simulink model "kwta2_block"  (R2024b)
settings: Solver=VariableStepAuto  StartTime=0.0  StopTime=2e-5  RelTol=1e-3
libraries: fl_lib x104, ee_lib x58, nesl_utility x13
(part 1 of 2)
settings Model: Creator=xyl  LastModifiedBy=James
settings SolverCC: AlgebraicLoopSolver=TrustRegion
settings DataIOCC: ReturnWorkspaceOutputs=off
settings DebuggingCC: UnconnectedInputMsg=warning  UnconnectedOutputMsg=warning  UnconnectedLineMsg=warning  ArithmeticOperatorsInVariantConditions=warning
settings ModelReferenceCC: EnableRefExpFcnMdlSchedulingChecks=on
settings SFSimCC: CustomCodeUndefinedFunction=UseInterfaceOnly
settings RTWCC: GPUComputeCapability=3.5

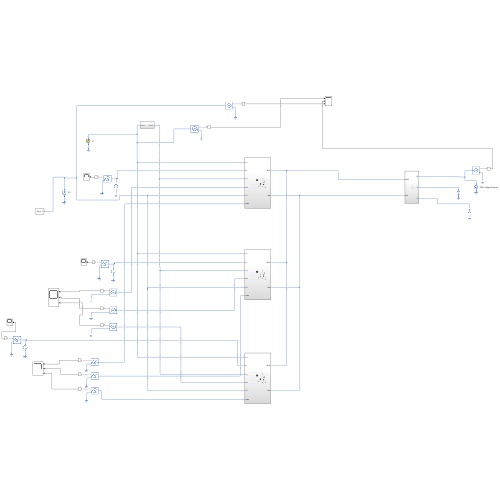
[thumbnail: Simulink's stored preview of the top-level diagram]
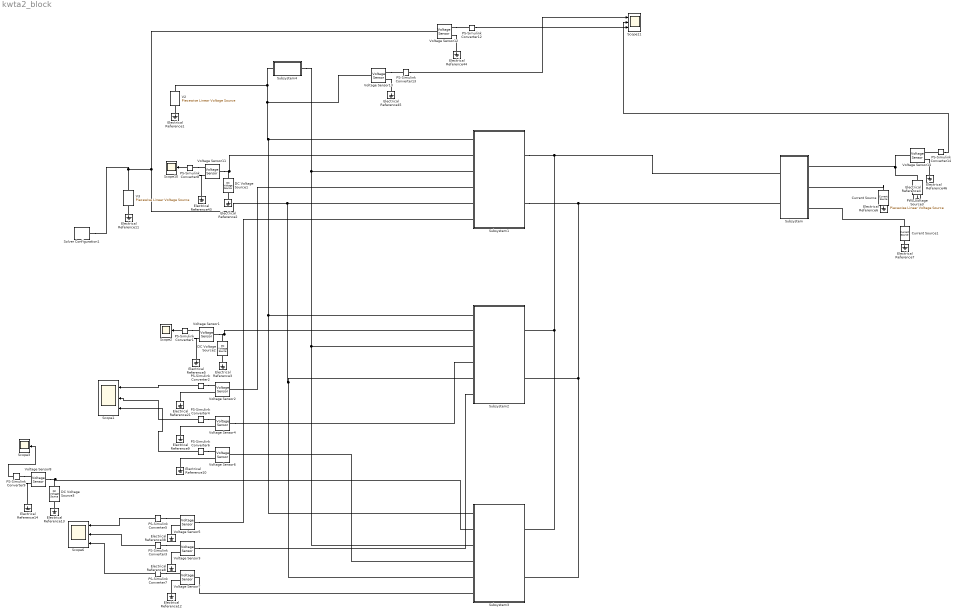
== system kwta2_block ==
  Current Source : ee_lib/Sources/Current Source  dc_current=40 uA  ac_current=0 A  ac_shift=0 rad  ac_frequency=60 Hz  noise_mode=0  PSD=0 A^2/Hz  sample_time=1e-3 s  repeatability=1  user_seed=0  auto_seed=3686359230  i_specify=off  i_priority=None  i=0 A  i_nominal_specify=off  i_nominal_value=1  i_nominal_unit=A  v_specify=off  v_priority=None  v=0 V  v_nominal_specify=off  v_nominal_value=1  v_nominal_unit=V
  Current Source1 : ee_lib/Sources/Current Source  dc_current=20 uA  ac_current=0 A  ac_shift=0 rad  ac_frequency=60 Hz  noise_mode=0  PSD=0 A^2/Hz  sample_time=1e-3 s  repeatability=1  user_seed=0  auto_seed=98181336  i_specify=off  i_priority=None  i=0 A  i_nominal_specify=off  i_nominal_value=1  i_nominal_unit=A  v_specify=off  v_priority=None  v=0 V  v_nominal_specify=off  v_nominal_value=1  v_nominal_unit=V
  DC Voltage Source1 : fl_lib/Electrical/Electrical Sources/DC Voltage Source  v0=0.1 V
  DC Voltage Source2 : fl_lib/Electrical/Electrical Sources/DC Voltage Source  v0=0.2 V
  DC Voltage Source3 : fl_lib/Electrical/Electrical Sources/DC Voltage Source  v0=0.3 V
  Electrical Reference{1..14,21,38,43..46} (20 alike) : fl_lib/Electrical/Electrical Elements/Electrical Reference
  PS-Simulink Converter{1..9,12..14} (12 alike) : nesl_utility/PS-Simulink Converter  PhysicalDomain=network_engine_domain  SubClassName=ps_output  LeftPortType=input  RightPortType=output  PseudoPeriodic=off  Frequencies=[]  VectorFormat=1-D array  Unit=1  AffineConversion=off
  PWL Voltage Source3 : ee_lib/Additional Components/SPICE Sources/Piecewise Linear Voltage Source  TIMElist=[0, 4, 4.01, 10, 10.01] us  VOLTlist=[0, 0, 5, 5, 5] V  INTERP=1  EXTRAP=2
      settings: InternalSimscapePortConfiguration="{\"Bottom\":[],\"Left\":[{\"id\":\"p\",\"label\":\"+\",\"type\":\"foundation.electrical.electrical\"}],\"Right\":[{\"id\":\"n\",\"label\":\"-\",\"type\":\"foundation.electrical.electrical\"}],\"Top\":[]}"
  Scope1 : Scope  NumInputPorts=3
  Scope10 : Scope
  Scope11 : Scope  NumInputPorts=3
  Scope2 : Scope
  Scope3 : Scope
  Scope6 : Scope  NumInputPorts=3
  Solver Configuration1 : nesl_utility/Solver Configuration  PhysicalDomain=network_engine_domain  SubClassName=solver  LeftPortType=input  RightPortType=generic  Tones=[]  Harmonics=[]  SimulateNoise=off  Profile=off  UseLocalSampling=off  EnableSwitchedLinearOptims=on  FrequencyDomain=off  UseCCode=off  RelTol=0.001  AbsTol=1e-06  MinStep=1e-09  ToWorkspace=off  RevertToSquareIcSolve=off  NumHomotopyIterations=100  PhasorMode=off  PhasorModeNumHarmonics=1  ConsistencySolver=NEWTON_FTOL  IndexReductionMethod=DerivativeReplacement  DoDC=on  ResidualTolerance=1e-09  ConsistencyTolSource=GLOBAL  ConsistencyAbsTol=0.001  ConsistencyRelTol=0.001  ConsistencyTolFactor=0.001  UseLocalSolver=on  LocalSolverChoice=NE_BACKWARD_EULER_ADVANCER  ResolveIndetEquations=on  FunctionEvalNumThread=1  LocalSolverSampleTime=1e-9  DoFixedCost=off  MaxNonlinIter=3  MaxModeIter=2  ComputeImpulses=off  ImpulseIterations=2  LinearAlgebra=Sparse  LinearAlgebraNumThread=0  EquationFormulation=NE_TIME_EF  DelaysMemoryBudget=1024  AutomaticFiltering=on  FilteringTimeConstant=0.01  PartitionStorageMethod=AS_NEEDED  PartitionMemoryBudget=1024  PartitionMethod=FAST  MultibodyUseLocalSolver=off  MultibodyLocalSolverChoice=ODE1  MultibodyLocalSolverSampleTime=0.001
  Subsystem : Subsystem
  Subsystem1 : Subsystem
  Subsystem2 : Subsystem
  Subsystem3 : Subsystem
  Subsystem4 : Subsystem
  V2 : ee_lib/Additional Components/SPICE Sources/Piecewise Linear Voltage Source  TIMElist=[0, 2, 2.01, 4, 4.1] us  VOLTlist=[0, 0, 5, 5, 5] V  INTERP=1  EXTRAP=2
      settings: InternalSimscapePortConfiguration="{\"Bottom\":[],\"Left\":[{\"id\":\"p\",\"label\":\"+\",\"type\":\"foundation.electrical.electrical\"}],\"Right\":[{\"id\":\"n\",\"label\":\"-\",\"type\":\"foundation.electrical.electrical\"}],\"Top\":[]}"
  V3 : ee_lib/Additional Components/SPICE Sources/Piecewise Linear Voltage Source  TIMElist=[0, 2, 14, 14.01, 16] us  VOLTlist=[0, 0, 0, 5, 5] V  INTERP=1  EXTRAP=2
      settings: InternalSimscapePortConfiguration="{\"Bottom\":[],\"Left\":[{\"id\":\"p\",\"label\":\"+\",\"type\":\"foundation.electrical.electrical\"}],\"Right\":[{\"id\":\"n\",\"label\":\"-\",\"type\":\"foundation.electrical.electrical\"}],\"Top\":[]}"
  Voltage Sensor{1..8,11..14} (12 alike) : fl_lib/Electrical/Electrical Sensors/Voltage Sensor
  wires:
  PS-Simulink Converter2/1 -> Scope1/1
  PS-Simulink Converter5/1 -> Scope6/1
  PS-Simulink Converter8/1 -> Scope10/1
  PS-Simulink Converter13/1 -> Scope11/1
  PS-Simulink Converter12/1 -> Scope11/3
  PS-Simulink Converter14/1 -> Scope11/2
  PS-Simulink Converter1/1 -> Scope2/1
  PS-Simulink Converter3/1 -> Scope6/2
  PS-Simulink Converter4/1 -> Scope1/2
  PS-Simulink Converter6/1 -> Scope1/3
  PS-Simulink Converter7/1 -> Scope6/3
  PS-Simulink Converter9/1 -> Scope3/1
  connections:
  Voltage Sensor11/LConn1 -- DC Voltage Source1/LConn1 -- Subsystem1/LConn2
  Electrical Reference1/LConn1 -- V2/RConn1
  Electrical Reference2/LConn1 -- DC Voltage Source1/RConn1
  Subsystem1/RConn1 -- Subsystem3/RConn1 -- Subsystem2/RConn1 -- Subsystem/LConn1
  Electrical Reference4/LConn1 -- PWL Voltage Source3/RConn1
  Electrical Reference6/LConn1 -- Current Source/RConn1
  Electrical Reference7/LConn1 -- Current Source1/RConn1
  Electrical Reference11/LConn1 -- V3/RConn1
  V3/LConn1 -- Solver Configuration1/RConn1 -- Voltage Sensor12/LConn1 -- Subsystem3/LConn5 -- Subsystem2/LConn5 -- Subsystem1/LConn5
  Voltage Sensor2/RConn2 -- Electrical Reference21/LConn1
  PS-Simulink Converter2/LConn1 -- Voltage Sensor2/RConn1
  Subsystem1/RConn2 -- Subsystem3/RConn2 -- Subsystem2/RConn2 -- Subsystem/LConn2
  Electrical Reference38/LConn1 -- Voltage Sensor5/RConn2
  PS-Simulink Converter5/LConn1 -- Voltage Sensor5/RConn1
  PS-Simulink Converter8/LConn1 -- Voltage Sensor11/RConn1
  Voltage Sensor11/RConn2 -- Electrical Reference43/LConn1
  Voltage Sensor12/RConn2 -- Electrical Reference44/LConn1
  Voltage Sensor12/RConn1 -- PS-Simulink Converter12/LConn1
  Voltage Sensor13/RConn2 -- Electrical Reference45/LConn1
  Voltage Sensor13/RConn1 -- PS-Simulink Converter13/LConn1
  Voltage Sensor14/RConn2 -- Electrical Reference46/LConn1
  PS-Simulink Converter14/LConn1 -- Voltage Sensor14/RConn1
  V2/LConn1 -- Subsystem4/RConn1 -- Subsystem3/LConn1 -- Subsystem2/LConn1 -- Subsystem1/LConn1 -- Voltage Sensor13/LConn1
  PWL Voltage Source3/LConn1 -- Voltage Sensor14/LConn1 -- Subsystem/RConn1
  Current Source/LConn1 -- Subsystem/RConn2
  Current Source1/LConn1 -- Subsystem/RConn3
  Subsystem4/LConn1 -- Subsystem3/LConn3 -- Subsystem2/LConn3 -- Subsystem1/LConn3
  Voltage Sensor5/LConn1 -- Subsystem1/LConn6
  Subsystem1/LConn4 -- Voltage Sensor2/LConn1
  Voltage Sensor1/LConn1 -- DC Voltage Source2/LConn1 -- Subsystem2/LConn2
  Voltage Sensor1/RConn2 -- Electrical Reference5/LConn1
  Electrical Reference3/LConn1 -- DC Voltage Source2/RConn1
  PS-Simulink Converter1/LConn1 -- Voltage Sensor1/RConn1
  PS-Simulink Converter3/LConn1 -- Voltage Sensor3/RConn1
  Electrical Reference8/LConn1 -- Voltage Sensor3/RConn2
  Voltage Sensor3/LConn1 -- Subsystem2/LConn6
  PS-Simulink Converter4/LConn1 -- Voltage Sensor4/RConn1
  Voltage Sensor4/RConn2 -- Electrical Reference9/LConn1
  Voltage Sensor4/LConn1 -- Subsystem2/LConn4
  Voltage Sensor6/RConn2 -- Electrical Reference10/LConn1
  PS-Simulink Converter6/LConn1 -- Voltage Sensor6/RConn1
  Subsystem3/LConn4 -- Voltage Sensor6/LConn1
  Subsystem3/LConn6 -- Voltage Sensor7/LConn1
  Electrical Reference12/LConn1 -- Voltage Sensor7/RConn2
  PS-Simulink Converter7/LConn1 -- Voltage Sensor7/RConn1
  DC Voltage Source3/LConn1 -- Subsystem3/LConn2 -- Voltage Sensor8/LConn1
  PS-Simulink Converter9/LConn1 -- Voltage Sensor8/RConn1
  Electrical Reference13/LConn1 -- DC Voltage Source3/RConn1
  Voltage Sensor8/RConn2 -- Electrical Reference14/LConn1

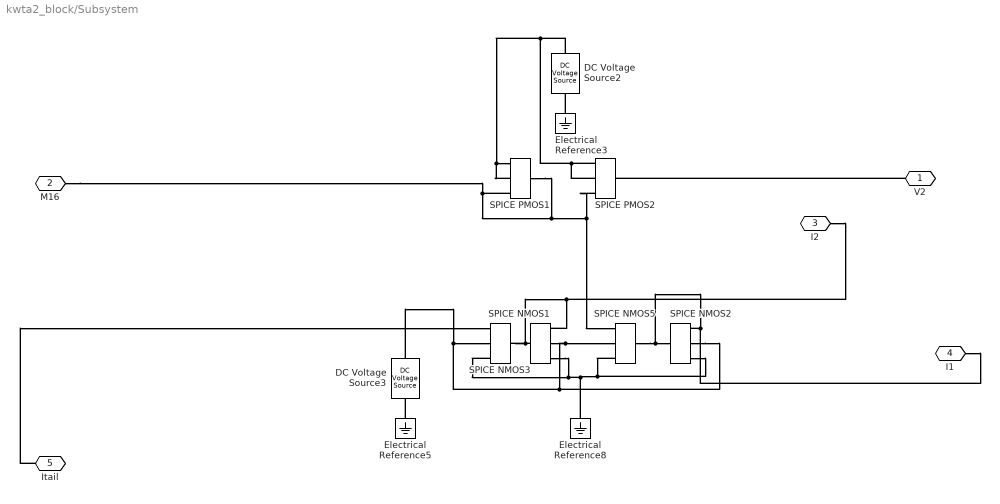
== system kwta2_block/Subsystem ==
  DC Voltage Source2 : fl_lib/Electrical/Electrical Sources/DC Voltage Source  v0=5 V
  DC Voltage Source3 : fl_lib/Electrical/Electrical Sources/DC Voltage Source  v0=-5 V
  Electrical Reference3 : fl_lib/Electrical/Electrical Elements/Electrical Reference
  Electrical Reference5 : fl_lib/Electrical/Electrical Elements/Electrical Reference
  Electrical Reference8 : fl_lib/Electrical/Electrical Elements/Electrical Reference
  SPICE NMOS{1..3,5} (4 alike) : ee_lib/Additional Components/SPICE Semiconductors/SPICE NMOS  LEVEL=3  AREA=1  SCALE=1  LENGTH=5 um  WIDTH=31 um  AD=0 m^2  AS=0 m^2  PD=0 m  PS=0 m  NRD=1  NRS=1  RD=0.01 Ohm  RS=1e-4 Ohm  RSH=NaN Ohm  VTO=0 V  KP=2e-5 A/V^2  GAMMA=0 V^0.50000  PHI=0.6 V  LAMBDA=0 1/V  IS=1e-14 A  N=1  JS=0 A/m^2  DELTA=0  VMAX=0 m/s  NFS=0 1/cm^2  ETA=0  THETA=0 1/V  KAPPA=0.2  Ci_param=ee.enum.intrinsicCapacitance.none  Cov_param=1  CGSO=0 F/m  CGDO=0 F/m  CGBO=0 F/m  C_param=1  CBD=0 F  CBS=0 F  PB=0.8 V  CJ=0 F/m^2  MJ=0.5  CJSW=0 F/m  MJSW=0.5  FC=0.5  IC_given=1  ICVDS=0 V  ICVGS=0 V  ICVBS=0 V  TOX=1e-7 m  LD=0 m  U0=600 cm^2/s/V  NSUB=NaN 1/cm^3  TPG=1  NSS=0 1/cm^2  XJ=0 m  T_param=1  TFIXED=300.15 K  TMEAS=300.15 K  TOFFSET=0 K  UEXP=0  UCRIT=1e+4 V/cm  NEFF=1  MTYPE=1
      settings: InternalSimscapePortConfiguration="{\"Bottom\":[],\"Left\":[{\"id\":\"gx\",\"label\":\"\",\"type\":\"foundation.electrical.electrical\"}],\"Right\":[{\"id\":\"dx\",\"label\":\"\",\"type\":\"foundation.electrical.electrical\"},{\"id\":\"bx\",\"label\":\"\",\"type\":\"foundation.electrical.electrical\"},{\"id\":\"sx\",\"label\":\"\",\"type\":\"foundation.electrical.electrical\"}],\"Top\":[]}"
  SPICE PMOS1 : ee_lib/Additional Components/SPICE Semiconductors/SPICE PMOS  LEVEL=3  AREA=1  SCALE=1  LENGTH=4 um  WIDTH=21 um  AD=0 m^2  AS=0 m^2  PD=0 m  PS=0 m  NRD=1  NRS=1  RD=0.01 Ohm  RS=1e-4 Ohm  RSH=NaN Ohm  VTO=0 V  KP=2e-5 A/V^2  GAMMA=0 V^0.50000  PHI=0.6 V  LAMBDA=0 1/V  IS=1e-14 A  N=1  JS=0 A/m^2  DELTA=0  VMAX=0 m/s  NFS=0 1/cm^2  ETA=0  THETA=0 1/V  KAPPA=0.2  Ci_param=ee.enum.intrinsicCapacitance.none  Cov_param=1  CGSO=0 F/m  CGDO=0 F/m  CGBO=0 F/m  C_param=1  CBD=0 F  CBS=0 F  PB=0.8 V  CJ=0 F/m^2  MJ=0.5  CJSW=0 F/m  MJSW=0.5  FC=0.5  IC_given=1  ICVDS=0 V  ICVGS=0 V  ICVBS=0 V  TOX=1e-7 m  LD=0 m  U0=600 cm^2/s/V  NSUB=NaN 1/cm^3  TPG=1  NSS=0 1/cm^2  XJ=0 m  T_param=1  TFIXED=300.15 K  TMEAS=300.15 K  TOFFSET=0 K  UEXP=0  UCRIT=1e+4 V/cm  NEFF=1  MTYPE=-1
      settings: InternalSimscapePortConfiguration="{\"Bottom\":[],\"Left\":[{\"id\":\"gx\",\"label\":\"\",\"type\":\"foundation.electrical.electrical\"}],\"Right\":[{\"id\":\"dx\",\"label\":\"\",\"type\":\"foundation.electrical.electrical\"},{\"id\":\"bx\",\"label\":\"\",\"type\":\"foundation.electrical.electrical\"},{\"id\":\"sx\",\"label\":\"\",\"type\":\"foundation.electrical.electrical\"}],\"Top\":[]}"
  SPICE PMOS2 : ee_lib/Additional Components/SPICE Semiconductors/SPICE PMOS  LEVEL=3  AREA=1  SCALE=1  LENGTH=5 um  WIDTH=31 um  AD=0 m^2  AS=0 m^2  PD=0 m  PS=0 m  NRD=1  NRS=1  RD=0.01 Ohm  RS=1e-4 Ohm  RSH=NaN Ohm  VTO=0 V  KP=2e-5 A/V^2  GAMMA=0 V^0.50000  PHI=0.6 V  LAMBDA=0 1/V  IS=1e-14 A  N=1  JS=0 A/m^2  DELTA=0  VMAX=0 m/s  NFS=0 1/cm^2  ETA=0  THETA=0 1/V  KAPPA=0.2  Ci_param=ee.enum.intrinsicCapacitance.none  Cov_param=1  CGSO=0 F/m  CGDO=0 F/m  CGBO=0 F/m  C_param=1  CBD=0 F  CBS=0 F  PB=0.8 V  CJ=0 F/m^2  MJ=0.5  CJSW=0 F/m  MJSW=0.5  FC=0.5  IC_given=1  ICVDS=0 V  ICVGS=0 V  ICVBS=0 V  TOX=1e-7 m  LD=0 m  U0=600 cm^2/s/V  NSUB=NaN 1/cm^3  TPG=1  NSS=0 1/cm^2  XJ=0 m  T_param=1  TFIXED=300.15 K  TMEAS=300.15 K  TOFFSET=0 K  UEXP=0  UCRIT=1e+4 V/cm  NEFF=1  MTYPE=-1
      settings: InternalSimscapePortConfiguration="{\"Bottom\":[],\"Left\":[{\"id\":\"gx\",\"label\":\"\",\"type\":\"foundation.electrical.electrical\"}],\"Right\":[{\"id\":\"dx\",\"label\":\"\",\"type\":\"foundation.electrical.electrical\"},{\"id\":\"bx\",\"label\":\"\",\"type\":\"foundation.electrical.electrical\"},{\"id\":\"sx\",\"label\":\"\",\"type\":\"foundation.electrical.electrical\"}],\"Top\":[]}"
  V2 : PMIOPort  Side=Right
  M16 : PMIOPort  Port=2  Side=Left
  I2 : PMIOPort  Port=3  Side=Right
  I1 : PMIOPort  Port=4  Side=Right
  Itail : PMIOPort  Port=5  Side=Left
  connections:
  SPICE PMOS1/LConn1 -- M16/RConn1 -- SPICE PMOS1/RConn1 -- SPICE PMOS2/RConn1 -- SPICE NMOS5/RConn1
  SPICE NMOS1/LConn1 -- I2/RConn1 -- SPICE NMOS1/RConn1 -- SPICE NMOS3/LConn1
  DC Voltage Source2/LConn1 -- SPICE PMOS2/RConn2 -- SPICE PMOS2/RConn3 -- SPICE PMOS1/RConn2 -- SPICE PMOS1/RConn3
  Itail/RConn1 -- SPICE NMOS3/RConn1
  V2/RConn1 -- SPICE PMOS2/LConn1
  SPICE NMOS1/RConn2 -- SPICE NMOS2/RConn2 -- DC Voltage Source3/LConn1 -- SPICE NMOS3/RConn2 -- SPICE NMOS5/RConn2
  SPICE NMOS5/LConn1 -- I1/RConn1 -- SPICE NMOS2/RConn1 -- SPICE NMOS2/LConn1
  Electrical Reference3/LConn1 -- DC Voltage Source2/RConn1
  Electrical Reference5/LConn1 -- DC Voltage Source3/RConn1
  Electrical Reference8/LConn1 -- SPICE NMOS2/RConn3 -- SPICE NMOS5/RConn3 -- SPICE NMOS3/RConn3 -- SPICE NMOS1/RConn3

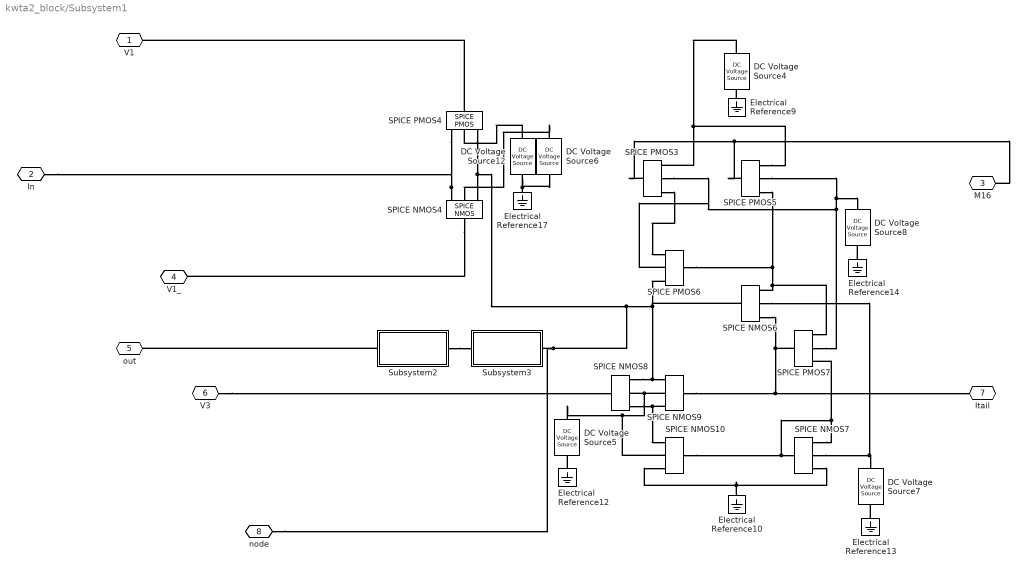
== system kwta2_block/Subsystem1 ==
  DC Voltage Source12 : fl_lib/Electrical/Electrical Sources/DC Voltage Source  v0=5 V
  DC Voltage Source4 : fl_lib/Electrical/Electrical Sources/DC Voltage Source  v0=5 V
  DC Voltage Source5 : fl_lib/Electrical/Electrical Sources/DC Voltage Source  v0=-5 V
  DC Voltage Source6 : fl_lib/Electrical/Electrical Sources/DC Voltage Source  v0=-5 V
  DC Voltage Source7 : fl_lib/Electrical/Electrical Sources/DC Voltage Source  v0=-5 V
  DC Voltage Source8 : fl_lib/Electrical/Electrical Sources/DC Voltage Source  v0=5 V
  Electrical Reference{9..10,12..14,17} (6 alike) : fl_lib/Electrical/Electrical Elements/Electrical Reference
  SPICE NMOS10 : ee_lib/Additional Components/SPICE Semiconductors/SPICE NMOS  LEVEL=3  AREA=1  SCALE=1  LENGTH=5 um  WIDTH=11 um  AD=0 m^2  AS=0 m^2  PD=0 m  PS=0 m  NRD=1  NRS=1  RD=0.01 Ohm  RS=1e-4 Ohm  RSH=NaN Ohm  VTO=0 V  KP=2e-5 A/V^2  GAMMA=0 V^0.50000  PHI=0.6 V  LAMBDA=0 1/V  IS=1e-14 A  N=1  JS=0 A/m^2  DELTA=0  VMAX=0 m/s  NFS=0 1/cm^2  ETA=0  THETA=0 1/V  KAPPA=0.2  Ci_param=ee.enum.intrinsicCapacitance.none  Cov_param=1  CGSO=0 F/m  CGDO=0 F/m  CGBO=0 F/m  C_param=1  CBD=0 F  CBS=0 F  PB=0.8 V  CJ=0 F/m^2  MJ=0.5  CJSW=0 F/m  MJSW=0.5  FC=0.5  IC_given=1  ICVDS=0 V  ICVGS=0 V  ICVBS=0 V  TOX=1e-7 m  LD=0 m  U0=600 cm^2/s/V  NSUB=NaN 1/cm^3  TPG=1  NSS=0 1/cm^2  XJ=0 m  T_param=1  TFIXED=300.15 K  TMEAS=300.15 K  TOFFSET=0 K  UEXP=0  UCRIT=1e+4 V/cm  NEFF=1  MTYPE=1
      settings: InternalSimscapePortConfiguration="{\"Bottom\":[],\"Left\":[{\"id\":\"gx\",\"label\":\"\",\"type\":\"foundation.electrical.electrical\"}],\"Right\":[{\"id\":\"dx\",\"label\":\"\",\"type\":\"foundation.electrical.electrical\"},{\"id\":\"bx\",\"label\":\"\",\"type\":\"foundation.electrical.electrical\"},{\"id\":\"sx\",\"label\":\"\",\"type\":\"foundation.electrical.electrical\"}],\"Top\":[]}"
  SPICE NMOS4 : ee_lib/Additional Components/SPICE Semiconductors/SPICE NMOS  LEVEL=3  AREA=1  SCALE=1  LENGTH=5 um  WIDTH=4 um  AD=0 m^2  AS=0 m^2  PD=0 m  PS=0 m  NRD=1  NRS=1  RD=0.01 Ohm  RS=1e-4 Ohm  RSH=NaN Ohm  VTO=0 V  KP=2e-5 A/V^2  GAMMA=0 V^0.50000  PHI=0.6 V  LAMBDA=0 1/V  IS=1e-14 A  N=1  JS=0 A/m^2  DELTA=0  VMAX=0 m/s  NFS=0 1/cm^2  ETA=0  THETA=0 1/V  KAPPA=0.2  Ci_param=ee.enum.intrinsicCapacitance.none  Cov_param=1  CGSO=0 F/m  CGDO=0 F/m  CGBO=0 F/m  C_param=1  CBD=0 F  CBS=0 F  PB=0.8 V  CJ=0 F/m^2  MJ=0.5  CJSW=0 F/m  MJSW=0.5  FC=0.5  IC_given=1  ICVDS=0 V  ICVGS=0 V  ICVBS=0 V  TOX=1e-7 m  LD=0 m  U0=600 cm^2/s/V  NSUB=NaN 1/cm^3  TPG=1  NSS=0 1/cm^2  XJ=0 m  T_param=1  TFIXED=300.15 K  TMEAS=300.15 K  TOFFSET=0 K  UEXP=0  UCRIT=1e+4 V/cm  NEFF=1  MTYPE=1
      settings: InternalSimscapePortConfiguration="{\"Bottom\":[],\"Left\":[{\"id\":\"gx\",\"label\":\"\",\"type\":\"foundation.electrical.electrical\"}],\"Right\":[{\"id\":\"dx\",\"label\":\"\",\"type\":\"foundation.electrical.electrical\"},{\"id\":\"bx\",\"label\":\"\",\"type\":\"foundation.electrical.electrical\"},{\"id\":\"sx\",\"label\":\"\",\"type\":\"foundation.electrical.electrical\"}],\"Top\":[]}"
  SPICE NMOS6 : ee_lib/Additional Components/SPICE Semiconductors/SPICE NMOS  LEVEL=3  AREA=1  SCALE=1  LENGTH=5 um  WIDTH=9 um  AD=0 m^2  AS=0 m^2  PD=0 m  PS=0 m  NRD=1  NRS=1  RD=0.01 Ohm  RS=1e-4 Ohm  RSH=NaN Ohm  VTO=0 V  KP=2e-5 A/V^2  GAMMA=0 V^0.50000  PHI=0.6 V  LAMBDA=0 1/V  IS=1e-14 A  N=1  JS=0 A/m^2  DELTA=0  VMAX=0 m/s  NFS=0 1/cm^2  ETA=0  THETA=0 1/V  KAPPA=0.2  Ci_param=ee.enum.intrinsicCapacitance.none  Cov_param=1  CGSO=0 F/m  CGDO=0 F/m  CGBO=0 F/m  C_param=1  CBD=0 F  CBS=0 F  PB=0.8 V  CJ=0 F/m^2  MJ=0.5  CJSW=0 F/m  MJSW=0.5  FC=0.5  IC_given=1  ICVDS=0 V  ICVGS=0 V  ICVBS=0 V  TOX=1e-7 m  LD=0 m  U0=600 cm^2/s/V  NSUB=NaN 1/cm^3  TPG=1  NSS=0 1/cm^2  XJ=0 m  T_param=1  TFIXED=300.15 K  TMEAS=300.15 K  TOFFSET=0 K  UEXP=0  UCRIT=1e+4 V/cm  NEFF=1  MTYPE=1
      settings: InternalSimscapePortConfiguration="{\"Bottom\":[],\"Left\":[{\"id\":\"gx\",\"label\":\"\",\"type\":\"foundation.electrical.electrical\"}],\"Right\":[{\"id\":\"dx\",\"label\":\"\",\"type\":\"foundation.electrical.electrical\"},{\"id\":\"bx\",\"label\":\"\",\"type\":\"foundation.electrical.electrical\"},{\"id\":\"sx\",\"label\":\"\",\"type\":\"foundation.electrical.electrical\"}],\"Top\":[]}"
  SPICE NMOS7 : ee_lib/Additional Components/SPICE Semiconductors/SPICE NMOS  LEVEL=3  AREA=1  SCALE=1  LENGTH=5 um  WIDTH=11 um  AD=0 m^2  AS=0 m^2  PD=0 m  PS=0 m  NRD=1  NRS=1  RD=0.01 Ohm  RS=1e-4 Ohm  RSH=NaN Ohm  VTO=0 V  KP=2e-5 A/V^2  GAMMA=0 V^0.50000  PHI=0.6 V  LAMBDA=0 1/V  IS=1e-14 A  N=1  JS=0 A/m^2  DELTA=0  VMAX=0 m/s  NFS=0 1/cm^2  ETA=0  THETA=0 1/V  KAPPA=0.2  Ci_param=ee.enum.intrinsicCapacitance.none  Cov_param=1  CGSO=0 F/m  CGDO=0 F/m  CGBO=0 F/m  C_param=1  CBD=0 F  CBS=0 F  PB=0.8 V  CJ=0 F/m^2  MJ=0.5  CJSW=0 F/m  MJSW=0.5  FC=0.5  IC_given=1  ICVDS=0 V  ICVGS=0 V  ICVBS=0 V  TOX=1e-7 m  LD=0 m  U0=600 cm^2/s/V  NSUB=NaN 1/cm^3  TPG=1  NSS=0 1/cm^2  XJ=0 m  T_param=1  TFIXED=300.15 K  TMEAS=300.15 K  TOFFSET=0 K  UEXP=0  UCRIT=1e+4 V/cm  NEFF=1  MTYPE=1
      settings: InternalSimscapePortConfiguration="{\"Bottom\":[],\"Left\":[{\"id\":\"gx\",\"label\":\"\",\"type\":\"foundation.electrical.electrical\"}],\"Right\":[{\"id\":\"dx\",\"label\":\"\",\"type\":\"foundation.electrical.electrical\"},{\"id\":\"bx\",\"label\":\"\",\"type\":\"foundation.electrical.electrical\"},{\"id\":\"sx\",\"label\":\"\",\"type\":\"foundation.electrical.electrical\"}],\"Top\":[]}"
  SPICE NMOS8 : ee_lib/Additional Components/SPICE Semiconductors/SPICE NMOS  LEVEL=3  AREA=1  SCALE=1  LENGTH=5 um  WIDTH=13 um  AD=0 m^2  AS=0 m^2  PD=0 m  PS=0 m  NRD=1  NRS=1  RD=0.01 Ohm  RS=1e-4 Ohm  RSH=NaN Ohm  VTO=0 V  KP=2e-5 A/V^2  GAMMA=0 V^0.50000  PHI=0.6 V  LAMBDA=0 1/V  IS=1e-14 A  N=1  JS=0 A/m^2  DELTA=0  VMAX=0 m/s  NFS=0 1/cm^2  ETA=0  THETA=0 1/V  KAPPA=0.2  Ci_param=ee.enum.intrinsicCapacitance.none  Cov_param=1  CGSO=0 F/m  CGDO=20 uF/m  CGBO=0 F/m  C_param=1  CBD=0 F  CBS=0 F  PB=0.8 V  CJ=0 F/m^2  MJ=0.5  CJSW=0 F/m  MJSW=0.5  FC=0.5  IC_given=1  ICVDS=0 V  ICVGS=0 V  ICVBS=0 V  TOX=1e-7 m  LD=0 m  U0=600 cm^2/s/V  NSUB=NaN 1/cm^3  TPG=1  NSS=0 1/cm^2  XJ=0 m  T_param=1  TFIXED=300.15 K  TMEAS=300.15 K  TOFFSET=0 K  UEXP=0  UCRIT=1e+4 V/cm  NEFF=1  MTYPE=1
      settings: InternalSimscapePortConfiguration="{\"Bottom\":[],\"Left\":[{\"id\":\"gx\",\"label\":\"\",\"type\":\"foundation.electrical.electrical\"}],\"Right\":[{\"id\":\"dx\",\"label\":\"\",\"type\":\"foundation.electrical.electrical\"},{\"id\":\"bx\",\"label\":\"\",\"type\":\"foundation.electrical.electrical\"},{\"id\":\"sx\",\"label\":\"\",\"type\":\"foundation.electrical.electrical\"}],\"Top\":[]}"
  SPICE NMOS9 : ee_lib/Additional Components/SPICE Semiconductors/SPICE NMOS  LEVEL=3  AREA=1  SCALE=1  LENGTH=5 um  WIDTH=13 um  AD=0 m^2  AS=0 m^2  PD=0 m  PS=0 m  NRD=1  NRS=1  RD=0.01 Ohm  RS=1e-4 Ohm  RSH=NaN Ohm  VTO=0 V  KP=2e-5 A/V^2  GAMMA=0 V^0.50000  PHI=0.6 V  LAMBDA=0 1/V  IS=1e-14 A  N=1  JS=0 A/m^2  DELTA=0  VMAX=0 m/s  NFS=0 1/cm^2  ETA=0  THETA=0 1/V  KAPPA=0.2  Ci_param=ee.enum.intrinsicCapacitance.none  Cov_param=2  CGSO=0 F/m  CGDO=1 uF/m  CGBO=0 F/m  C_param=2  CBD=0 F  CBS=0 F  PB=0.8 V  CJ=0 F/m^2  MJ=0.5  CJSW=0 F/m  MJSW=0.5  FC=0.5  IC_given=1  ICVDS=0 V  ICVGS=0 V  ICVBS=0 V  TOX=1e-7 m  LD=0 m  U0=600 cm^2/s/V  NSUB=NaN 1/cm^3  TPG=1  NSS=0 1/cm^2  XJ=0 m  T_param=1  TFIXED=300.15 K  TMEAS=300.15 K  TOFFSET=0 K  UEXP=0  UCRIT=1e+4 V/cm  NEFF=1  MTYPE=1
      settings: InternalSimscapePortConfiguration="{\"Bottom\":[],\"Left\":[{\"id\":\"gx\",\"label\":\"\",\"type\":\"foundation.electrical.electrical\"}],\"Right\":[{\"id\":\"dx\",\"label\":\"\",\"type\":\"foundation.electrical.electrical\"},{\"id\":\"bx\",\"label\":\"\",\"type\":\"foundation.electrical.electrical\"},{\"id\":\"sx\",\"label\":\"\",\"type\":\"foundation.electrical.electrical\"}],\"Top\":[]}"
  SPICE PMOS3 : ee_lib/Additional Components/SPICE Semiconductors/SPICE PMOS  LEVEL=3  AREA=1  SCALE=1  LENGTH=4 um  WIDTH=7 um  AD=0 m^2  AS=0 m^2  PD=0 m  PS=0 m  NRD=1  NRS=1  RD=0.01 Ohm  RS=1e-4 Ohm  RSH=NaN Ohm  VTO=0 V  KP=2e-5 A/V^2  GAMMA=0 V^0.50000  PHI=0.6 V  LAMBDA=0 1/V  IS=1e-14 A  N=1  JS=0 A/m^2  DELTA=0  VMAX=0 m/s  NFS=0 1/cm^2  ETA=0  THETA=0 1/V  KAPPA=0.2  Ci_param=ee.enum.intrinsicCapacitance.none  Cov_param=1  CGSO=0 F/m  CGDO=0 F/m  CGBO=0 F/m  C_param=1  CBD=0 F  CBS=0 F  PB=0.8 V  CJ=0 F/m^2  MJ=0.5  CJSW=0 F/m  MJSW=0.5  FC=0.5  IC_given=1  ICVDS=0 V  ICVGS=0 V  ICVBS=0 V  TOX=1e-7 m  LD=0 m  U0=600 cm^2/s/V  NSUB=NaN 1/cm^3  TPG=1  NSS=0 1/cm^2  XJ=0 m  T_param=1  TFIXED=300.15 K  TMEAS=300.15 K  TOFFSET=0 K  UEXP=0  UCRIT=1e+4 V/cm  NEFF=1  MTYPE=-1
      settings: InternalSimscapePortConfiguration="{\"Bottom\":[],\"Left\":[{\"id\":\"gx\",\"label\":\"\",\"type\":\"foundation.electrical.electrical\"}],\"Right\":[{\"id\":\"dx\",\"label\":\"\",\"type\":\"foundation.electrical.electrical\"},{\"id\":\"bx\",\"label\":\"\",\"type\":\"foundation.electrical.electrical\"},{\"id\":\"sx\",\"label\":\"\",\"type\":\"foundation.electrical.electrical\"}],\"Top\":[]}"
  SPICE PMOS4 : ee_lib/Additional Components/SPICE Semiconductors/SPICE PMOS  LEVEL=3  AREA=1  SCALE=1  LENGTH=5 um  WIDTH=4 um  AD=0 m^2  AS=0 m^2  PD=0 m  PS=0 m  NRD=1  NRS=1  RD=0.01 Ohm  RS=1e-4 Ohm  RSH=NaN Ohm  VTO=0 V  KP=2e-5 A/V^2  GAMMA=0 V^0.50000  PHI=0.6 V  LAMBDA=0 1/V  IS=1e-14 A  N=1  JS=0 A/m^2  DELTA=0  VMAX=0 m/s  NFS=0 1/cm^2  ETA=0  THETA=0 1/V  KAPPA=0.2  Ci_param=ee.enum.intrinsicCapacitance.none  Cov_param=1  CGSO=0 F/m  CGDO=0 F/m  CGBO=0 F/m  C_param=1  CBD=0 F  CBS=0 F  PB=0.8 V  CJ=0 F/m^2  MJ=0.5  CJSW=0 F/m  MJSW=0.5  FC=0.5  IC_given=1  ICVDS=0 V  ICVGS=0 V  ICVBS=0 V  TOX=1e-7 m  LD=0 m  U0=600 cm^2/s/V  NSUB=NaN 1/cm^3  TPG=1  NSS=0 1/cm^2  XJ=0 m  T_param=1  TFIXED=300.15 K  TMEAS=300.15 K  TOFFSET=0 K  UEXP=0  UCRIT=1e+4 V/cm  NEFF=1  MTYPE=-1
      settings: InternalSimscapePortConfiguration="{\"Bottom\":[],\"Left\":[{\"id\":\"gx\",\"label\":\"\",\"type\":\"foundation.electrical.electrical\"}],\"Right\":[{\"id\":\"dx\",\"label\":\"\",\"type\":\"foundation.electrical.electrical\"},{\"id\":\"bx\",\"label\":\"\",\"type\":\"foundation.electrical.electrical\"},{\"id\":\"sx\",\"label\":\"\",\"type\":\"foundation.electrical.electrical\"}],\"Top\":[]}"
  SPICE PMOS5 : ee_lib/Additional Components/SPICE Semiconductors/SPICE PMOS  LEVEL=3  AREA=1  SCALE=1  LENGTH=4 um  WIDTH=21 um  AD=0 m^2  AS=0 m^2  PD=0 m  PS=0 m  NRD=1  NRS=1  RD=0.01 Ohm  RS=1e-4 Ohm  RSH=NaN Ohm  VTO=0 V  KP=2e-5 A/V^2  GAMMA=0 V^0.50000  PHI=0.6 V  LAMBDA=0 1/V  IS=1e-14 A  N=1  JS=0 A/m^2  DELTA=0  VMAX=0 m/s  NFS=0 1/cm^2  ETA=0  THETA=0 1/V  KAPPA=0.2  Ci_param=ee.enum.intrinsicCapacitance.none  Cov_param=1  CGSO=0 F/m  CGDO=0 F/m  CGBO=0 F/m  C_param=1  CBD=0 F  CBS=0 F  PB=0.8 V  CJ=0 F/m^2  MJ=0.5  CJSW=0 F/m  MJSW=0.5  FC=0.5  IC_given=1  ICVDS=0 V  ICVGS=0 V  ICVBS=0 V  TOX=1e-7 m  LD=0 m  U0=600 cm^2/s/V  NSUB=NaN 1/cm^3  TPG=1  NSS=0 1/cm^2  XJ=0 m  T_param=1  TFIXED=300.15 K  TMEAS=300.15 K  TOFFSET=0 K  UEXP=0  UCRIT=1e+4 V/cm  NEFF=1  MTYPE=-1
      settings: InternalSimscapePortConfiguration="{\"Bottom\":[],\"Left\":[{\"id\":\"gx\",\"label\":\"\",\"type\":\"foundation.electrical.electrical\"}],\"Right\":[{\"id\":\"dx\",\"label\":\"\",\"type\":\"foundation.electrical.electrical\"},{\"id\":\"bx\",\"label\":\"\",\"type\":\"foundation.electrical.electrical\"},{\"id\":\"sx\",\"label\":\"\",\"type\":\"foundation.electrical.electrical\"}],\"Top\":[]}"
  SPICE PMOS6 : ee_lib/Additional Components/SPICE Semiconductors/SPICE PMOS  LEVEL=3  AREA=1  SCALE=1  LENGTH=4 um  WIDTH=7 um  AD=0 m^2  AS=0 m^2  PD=0 m  PS=0 m  NRD=1  NRS=1  RD=0.01 Ohm  RS=1e-4 Ohm  RSH=NaN Ohm  VTO=0 V  KP=2e-5 A/V^2  GAMMA=0 V^0.50000  PHI=0.6 V  LAMBDA=0 1/V  IS=1e-14 A  N=1  JS=0 A/m^2  DELTA=0  VMAX=0 m/s  NFS=0 1/cm^2  ETA=0  THETA=0 1/V  KAPPA=0.2  Ci_param=ee.enum.intrinsicCapacitance.none  Cov_param=1  CGSO=0 F/m  CGDO=0 F/m  CGBO=0 F/m  C_param=1  CBD=0 F  CBS=0 F  PB=0.8 V  CJ=0 F/m^2  MJ=0.5  CJSW=0 F/m  MJSW=0.5  FC=0.5  IC_given=1  ICVDS=0 V  ICVGS=0 V  ICVBS=0 V  TOX=1e-7 m  LD=0 m  U0=600 cm^2/s/V  NSUB=NaN 1/cm^3  TPG=1  NSS=0 1/cm^2  XJ=0 m  T_param=1  TFIXED=300.15 K  TMEAS=300.15 K  TOFFSET=0 K  UEXP=0  UCRIT=1e+4 V/cm  NEFF=1  MTYPE=-1
      settings: InternalSimscapePortConfiguration="{\"Bottom\":[],\"Left\":[{\"id\":\"gx\",\"label\":\"\",\"type\":\"foundation.electrical.electrical\"}],\"Right\":[{\"id\":\"dx\",\"label\":\"\",\"type\":\"foundation.electrical.electrical\"},{\"id\":\"bx\",\"label\":\"\",\"type\":\"foundation.electrical.electrical\"},{\"id\":\"sx\",\"label\":\"\",\"type\":\"foundation.electrical.electrical\"}],\"Top\":[]}"
  SPICE PMOS7 : ee_lib/Additional Components/SPICE Semiconductors/SPICE PMOS  LEVEL=3  AREA=1  SCALE=1  LENGTH=4 um  WIDTH=17 um  AD=0 m^2  AS=0 m^2  PD=0 m  PS=0 m  NRD=1  NRS=1  RD=0.01 Ohm  RS=1e-4 Ohm  RSH=NaN Ohm  VTO=0 V  KP=2e-5 A/V^2  GAMMA=0 V^0.50000  PHI=0.6 V  LAMBDA=0 1/V  IS=1e-14 A  N=1  JS=0 A/m^2  DELTA=0  VMAX=0 m/s  NFS=0 1/cm^2  ETA=0  THETA=0 1/V  KAPPA=0.2  Ci_param=ee.enum.intrinsicCapacitance.none  Cov_param=1  CGSO=0 F/m  CGDO=0 F/m  CGBO=0 F/m  C_param=1  CBD=0 F  CBS=0 F  PB=0.8 V  CJ=0 F/m^2  MJ=0.5  CJSW=0 F/m  MJSW=0.5  FC=0.5  IC_given=1  ICVDS=0 V  ICVGS=0 V  ICVBS=0 V  TOX=1e-7 m  LD=0 m  U0=600 cm^2/s/V  NSUB=NaN 1/cm^3  TPG=1  NSS=0 1/cm^2  XJ=0 m  T_param=1  TFIXED=300.15 K  TMEAS=300.15 K  TOFFSET=0 K  UEXP=0  UCRIT=1e+4 V/cm  NEFF=1  MTYPE=-1
      settings: InternalSimscapePortConfiguration="{\"Bottom\":[],\"Left\":[{\"id\":\"gx\",\"label\":\"\",\"type\":\"foundation.electrical.electrical\"}],\"Right\":[{\"id\":\"dx\",\"label\":\"\",\"type\":\"foundation.electrical.electrical\"},{\"id\":\"bx\",\"label\":\"\",\"type\":\"foundation.electrical.electrical\"},{\"id\":\"sx\",\"label\":\"\",\"type\":\"foundation.electrical.electrical\"}],\"Top\":[]}"
  Subsystem2 : Subsystem
  Subsystem3 : Subsystem
  V1 : PMIOPort  Side=Left
  In : PMIOPort  Port=2  Side=Left
  M16 : PMIOPort  Port=3  Side=Right
  V1_ : PMIOPort  Port=4  Side=Left
  out : PMIOPort  Port=5  Side=Left
  V3 : PMIOPort  Port=6  Side=Left
  Itail : PMIOPort  Port=7  Side=Right
  "node " : PMIOPort  Port=8  Side=Left
  connections:
  SPICE NMOS6/RConn3 -- Itail/RConn1 -- SPICE NMOS9/LConn1 -- SPICE PMOS7/LConn1
  SPICE PMOS5/RConn3 -- SPICE PMOS6/LConn1 -- SPICE PMOS7/RConn1 -- SPICE NMOS6/RConn1
  Electrical Reference10/LConn1 -- SPICE NMOS10/RConn3 -- SPICE NMOS7/RConn3
  Subsystem2/LConn1 -- out/RConn1
  DC Voltage Source4/LConn1 -- SPICE PMOS3/RConn1 -- SPICE PMOS5/RConn1
  DC Voltage Source6/LConn1 -- SPICE NMOS4/RConn2
  V3/RConn1 -- SPICE NMOS8/LConn1
  DC Voltage Source12/LConn1 -- SPICE PMOS4/RConn2
  DC Voltage Source5/LConn1 -- SPICE NMOS10/RConn2 -- SPICE NMOS9/RConn2 -- SPICE NMOS8/RConn2
  DC Voltage Source12/RConn1 -- DC Voltage Source6/RConn1 -- Electrical Reference17/LConn1
  SPICE NMOS4/RConn1 -- SPICE PMOS4/RConn3 -- In/RConn1
  SPICE PMOS5/LConn1 -- M16/RConn1 -- SPICE PMOS3/LConn1
  SPICE PMOS4/LConn1 -- V1/RConn1
  Electrical Reference9/LConn1 -- DC Voltage Source4/RConn1
  Electrical Reference14/LConn1 -- DC Voltage Source8/RConn1
  SPICE PMOS7/RConn2 -- SPICE PMOS3/RConn2 -- SPICE PMOS6/RConn2 -- SPICE PMOS5/RConn2 -- DC Voltage Source8/LConn1
  SPICE PMOS3/RConn3 -- SPICE PMOS6/RConn1
  SPICE NMOS10/LConn1 -- SPICE PMOS7/RConn3 -- SPICE NMOS7/RConn1 -- SPICE NMOS7/LConn1
  SPICE PMOS4/RConn1 -- SPICE NMOS4/RConn3 -- "node "/RConn1 -- Subsystem3/RConn1 -- SPICE PMOS6/RConn3 -- SPICE NMOS6/LConn1 -- SPICE NMOS8/RConn1 -- SPICE NMOS9/RConn1
  SPICE NMOS7/RConn2 -- SPICE NMOS6/RConn2 -- DC Voltage Source7/LConn1
  SPICE NMOS9/RConn3 -- SPICE NMOS8/RConn3 -- SPICE NMOS10/RConn1
  Subsystem2/RConn1 -- Subsystem3/LConn1
  SPICE NMOS4/LConn1 -- V1_/RConn1
  Electrical Reference13/LConn1 -- DC Voltage Source7/RConn1
  Electrical Reference12/LConn1 -- DC Voltage Source5/RConn1

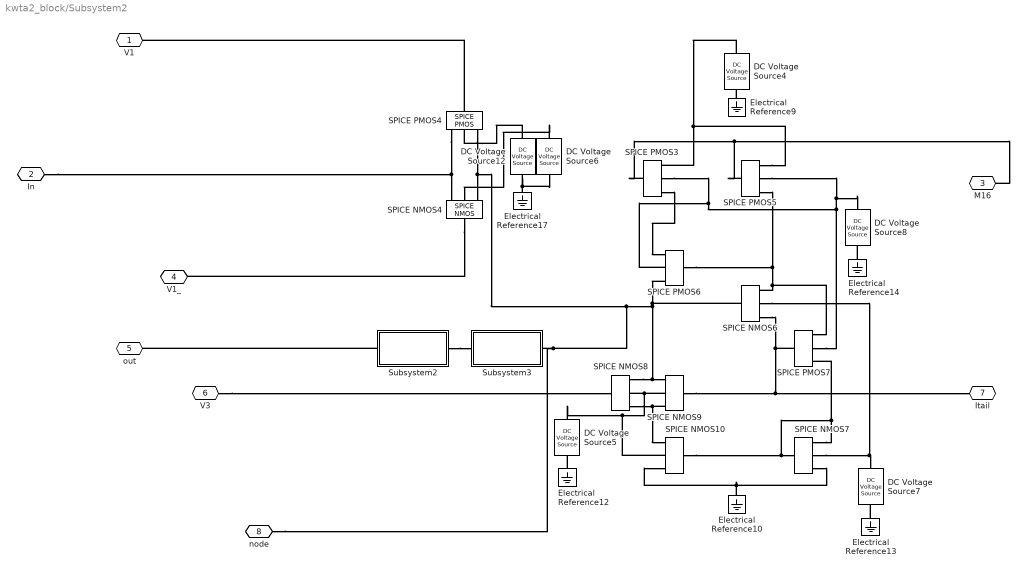
== system kwta2_block/Subsystem2 ==
  DC Voltage Source12 : fl_lib/Electrical/Electrical Sources/DC Voltage Source  v0=5 V
  DC Voltage Source4 : fl_lib/Electrical/Electrical Sources/DC Voltage Source  v0=5 V
  DC Voltage Source5 : fl_lib/Electrical/Electrical Sources/DC Voltage Source  v0=-5 V
  DC Voltage Source6 : fl_lib/Electrical/Electrical Sources/DC Voltage Source  v0=-5 V
  DC Voltage Source7 : fl_lib/Electrical/Electrical Sources/DC Voltage Source  v0=-5 V
  DC Voltage Source8 : fl_lib/Electrical/Electrical Sources/DC Voltage Source  v0=5 V
  Electrical Reference{9..10,12..14,17} (6 alike) : fl_lib/Electrical/Electrical Elements/Electrical Reference
  SPICE NMOS10 : ee_lib/Additional Components/SPICE Semiconductors/SPICE NMOS  LEVEL=3  AREA=1  SCALE=1  LENGTH=5 um  WIDTH=11 um  AD=0 m^2  AS=0 m^2  PD=0 m  PS=0 m  NRD=1  NRS=1  RD=0.01 Ohm  RS=1e-4 Ohm  RSH=NaN Ohm  VTO=0 V  KP=2e-5 A/V^2  GAMMA=0 V^0.50000  PHI=0.6 V  LAMBDA=0 1/V  IS=1e-14 A  N=1  JS=0 A/m^2  DELTA=0  VMAX=0 m/s  NFS=0 1/cm^2  ETA=0  THETA=0 1/V  KAPPA=0.2  Ci_param=ee.enum.intrinsicCapacitance.none  Cov_param=1  CGSO=0 F/m  CGDO=0 F/m  CGBO=0 F/m  C_param=1  CBD=0 F  CBS=0 F  PB=0.8 V  CJ=0 F/m^2  MJ=0.5  CJSW=0 F/m  MJSW=0.5  FC=0.5  IC_given=1  ICVDS=0 V  ICVGS=0 V  ICVBS=0 V  TOX=1e-7 m  LD=0 m  U0=600 cm^2/s/V  NSUB=NaN 1/cm^3  TPG=1  NSS=0 1/cm^2  XJ=0 m  T_param=1  TFIXED=300.15 K  TMEAS=300.15 K  TOFFSET=0 K  UEXP=0  UCRIT=1e+4 V/cm  NEFF=1  MTYPE=1
      settings: InternalSimscapePortConfiguration="{\"Bottom\":[],\"Left\":[{\"id\":\"gx\",\"label\":\"\",\"type\":\"foundation.electrical.electrical\"}],\"Right\":[{\"id\":\"dx\",\"label\":\"\",\"type\":\"foundation.electrical.electrical\"},{\"id\":\"bx\",\"label\":\"\",\"type\":\"foundation.electrical.electrical\"},{\"id\":\"sx\",\"label\":\"\",\"type\":\"foundation.electrical.electrical\"}],\"Top\":[]}"
  SPICE NMOS4 : ee_lib/Additional Components/SPICE Semiconductors/SPICE NMOS  LEVEL=3  AREA=1  SCALE=1  LENGTH=5 um  WIDTH=4 um  AD=0 m^2  AS=0 m^2  PD=0 m  PS=0 m  NRD=1  NRS=1  RD=0.01 Ohm  RS=1e-4 Ohm  RSH=NaN Ohm  VTO=0 V  KP=2e-5 A/V^2  GAMMA=0 V^0.50000  PHI=0.6 V  LAMBDA=0 1/V  IS=1e-14 A  N=1  JS=0 A/m^2  DELTA=0  VMAX=0 m/s  NFS=0 1/cm^2  ETA=0  THETA=0 1/V  KAPPA=0.2  Ci_param=ee.enum.intrinsicCapacitance.none  Cov_param=1  CGSO=0 F/m  CGDO=0 F/m  CGBO=0 F/m  C_param=1  CBD=0 F  CBS=0 F  PB=0.8 V  CJ=0 F/m^2  MJ=0.5  CJSW=0 F/m  MJSW=0.5  FC=0.5  IC_given=1  ICVDS=0 V  ICVGS=0 V  ICVBS=0 V  TOX=1e-7 m  LD=0 m  U0=600 cm^2/s/V  NSUB=NaN 1/cm^3  TPG=1  NSS=0 1/cm^2  XJ=0 m  T_param=1  TFIXED=300.15 K  TMEAS=300.15 K  TOFFSET=0 K  UEXP=0  UCRIT=1e+4 V/cm  NEFF=1  MTYPE=1
      settings: InternalSimscapePortConfiguration="{\"Bottom\":[],\"Left\":[{\"id\":\"gx\",\"label\":\"\",\"type\":\"foundation.electrical.electrical\"}],\"Right\":[{\"id\":\"dx\",\"label\":\"\",\"type\":\"foundation.electrical.electrical\"},{\"id\":\"bx\",\"label\":\"\",\"type\":\"foundation.electrical.electrical\"},{\"id\":\"sx\",\"label\":\"\",\"type\":\"foundation.electrical.electrical\"}],\"Top\":[]}"
  SPICE NMOS6 : ee_lib/Additional Components/SPICE Semiconductors/SPICE NMOS  LEVEL=3  AREA=1  SCALE=1  LENGTH=5 um  WIDTH=9 um  AD=0 m^2  AS=0 m^2  PD=0 m  PS=0 m  NRD=1  NRS=1  RD=0.01 Ohm  RS=1e-4 Ohm  RSH=NaN Ohm  VTO=0 V  KP=2e-5 A/V^2  GAMMA=0 V^0.50000  PHI=0.6 V  LAMBDA=0 1/V  IS=1e-14 A  N=1  JS=0 A/m^2  DELTA=0  VMAX=0 m/s  NFS=0 1/cm^2  ETA=0  THETA=0 1/V  KAPPA=0.2  Ci_param=ee.enum.intrinsicCapacitance.none  Cov_param=1  CGSO=0 F/m  CGDO=0 F/m  CGBO=0 F/m  C_param=1  CBD=0 F  CBS=0 F  PB=0.8 V  CJ=0 F/m^2  MJ=0.5  CJSW=0 F/m  MJSW=0.5  FC=0.5  IC_given=1  ICVDS=0 V  ICVGS=0 V  ICVBS=0 V  TOX=1e-7 m  LD=0 m  U0=600 cm^2/s/V  NSUB=NaN 1/cm^3  TPG=1  NSS=0 1/cm^2  XJ=0 m  T_param=1  TFIXED=300.15 K  TMEAS=300.15 K  TOFFSET=0 K  UEXP=0  UCRIT=1e+4 V/cm  NEFF=1  MTYPE=1
      settings: InternalSimscapePortConfiguration="{\"Bottom\":[],\"Left\":[{\"id\":\"gx\",\"label\":\"\",\"type\":\"foundation.electrical.electrical\"}],\"Right\":[{\"id\":\"dx\",\"label\":\"\",\"type\":\"foundation.electrical.electrical\"},{\"id\":\"bx\",\"label\":\"\",\"type\":\"foundation.electrical.electrical\"},{\"id\":\"sx\",\"label\":\"\",\"type\":\"foundation.electrical.electrical\"}],\"Top\":[]}"
  SPICE NMOS7 : ee_lib/Additional Components/SPICE Semiconductors/SPICE NMOS  LEVEL=3  AREA=1  SCALE=1  LENGTH=5 um  WIDTH=11 um  AD=0 m^2  AS=0 m^2  PD=0 m  PS=0 m  NRD=1  NRS=1  RD=0.01 Ohm  RS=1e-4 Ohm  RSH=NaN Ohm  VTO=0 V  KP=2e-5 A/V^2  GAMMA=0 V^0.50000  PHI=0.6 V  LAMBDA=0 1/V  IS=1e-14 A  N=1  JS=0 A/m^2  DELTA=0  VMAX=0 m/s  NFS=0 1/cm^2  ETA=0  THETA=0 1/V  KAPPA=0.2  Ci_param=ee.enum.intrinsicCapacitance.none  Cov_param=1  CGSO=0 F/m  CGDO=0 F/m  CGBO=0 F/m  C_param=1  CBD=0 F  CBS=0 F  PB=0.8 V  CJ=0 F/m^2  MJ=0.5  CJSW=0 F/m  MJSW=0.5  FC=0.5  IC_given=1  ICVDS=0 V  ICVGS=0 V  ICVBS=0 V  TOX=1e-7 m  LD=0 m  U0=600 cm^2/s/V  NSUB=NaN 1/cm^3  TPG=1  NSS=0 1/cm^2  XJ=0 m  T_param=1  TFIXED=300.15 K  TMEAS=300.15 K  TOFFSET=0 K  UEXP=0  UCRIT=1e+4 V/cm  NEFF=1  MTYPE=1
      settings: InternalSimscapePortConfiguration="{\"Bottom\":[],\"Left\":[{\"id\":\"gx\",\"label\":\"\",\"type\":\"foundation.electrical.electrical\"}],\"Right\":[{\"id\":\"dx\",\"label\":\"\",\"type\":\"foundation.electrical.electrical\"},{\"id\":\"bx\",\"label\":\"\",\"type\":\"foundation.electrical.electrical\"},{\"id\":\"sx\",\"label\":\"\",\"type\":\"foundation.electrical.electrical\"}],\"Top\":[]}"
  SPICE NMOS8 : ee_lib/Additional Components/SPICE Semiconductors/SPICE NMOS  LEVEL=3  AREA=1  SCALE=1  LENGTH=5 um  WIDTH=13 um  AD=0 m^2  AS=0 m^2  PD=0 m  PS=0 m  NRD=1  NRS=1  RD=0.01 Ohm  RS=1e-4 Ohm  RSH=NaN Ohm  VTO=0 V  KP=2e-5 A/V^2  GAMMA=0 V^0.50000  PHI=0.6 V  LAMBDA=0 1/V  IS=1e-14 A  N=1  JS=0 A/m^2  DELTA=0  VMAX=0 m/s  NFS=0 1/cm^2  ETA=0  THETA=0 1/V  KAPPA=0.2  Ci_param=ee.enum.intrinsicCapacitance.none  Cov_param=1  CGSO=0 F/m  CGDO=20 uF/m  CGBO=0 F/m  C_param=1  CBD=0 F  CBS=0 F  PB=0.8 V  CJ=0 F/m^2  MJ=0.5  CJSW=0 F/m  MJSW=0.5  FC=0.5  IC_given=1  ICVDS=0 V  ICVGS=0 V  ICVBS=0 V  TOX=1e-7 m  LD=0 m  U0=600 cm^2/s/V  NSUB=NaN 1/cm^3  TPG=1  NSS=0 1/cm^2  XJ=0 m  T_param=1  TFIXED=300.15 K  TMEAS=300.15 K  TOFFSET=0 K  UEXP=0  UCRIT=1e+4 V/cm  NEFF=1  MTYPE=1
      settings: InternalSimscapePortConfiguration="{\"Bottom\":[],\"Left\":[{\"id\":\"gx\",\"label\":\"\",\"type\":\"foundation.electrical.electrical\"}],\"Right\":[{\"id\":\"dx\",\"label\":\"\",\"type\":\"foundation.electrical.electrical\"},{\"id\":\"bx\",\"label\":\"\",\"type\":\"foundation.electrical.electrical\"},{\"id\":\"sx\",\"label\":\"\",\"type\":\"foundation.electrical.electrical\"}],\"Top\":[]}"
  SPICE NMOS9 : ee_lib/Additional Components/SPICE Semiconductors/SPICE NMOS  LEVEL=3  AREA=1  SCALE=1  LENGTH=5 um  WIDTH=13 um  AD=0 m^2  AS=0 m^2  PD=0 m  PS=0 m  NRD=1  NRS=1  RD=0.01 Ohm  RS=1e-4 Ohm  RSH=NaN Ohm  VTO=0 V  KP=2e-5 A/V^2  GAMMA=0 V^0.50000  PHI=0.6 V  LAMBDA=0 1/V  IS=1e-14 A  N=1  JS=0 A/m^2  DELTA=0  VMAX=0 m/s  NFS=0 1/cm^2  ETA=0  THETA=0 1/V  KAPPA=0.2  Ci_param=ee.enum.intrinsicCapacitance.none  Cov_param=2  CGSO=0 F/m  CGDO=1 uF/m  CGBO=0 F/m  C_param=2  CBD=0 F  CBS=0 F  PB=0.8 V  CJ=0 F/m^2  MJ=0.5  CJSW=0 F/m  MJSW=0.5  FC=0.5  IC_given=1  ICVDS=0 V  ICVGS=0 V  ICVBS=0 V  TOX=1e-7 m  LD=0 m  U0=600 cm^2/s/V  NSUB=NaN 1/cm^3  TPG=1  NSS=0 1/cm^2  XJ=0 m  T_param=1  TFIXED=300.15 K  TMEAS=300.15 K  TOFFSET=0 K  UEXP=0  UCRIT=1e+4 V/cm  NEFF=1  MTYPE=1
      settings: InternalSimscapePortConfiguration="{\"Bottom\":[],\"Left\":[{\"id\":\"gx\",\"label\":\"\",\"type\":\"foundation.electrical.electrical\"}],\"Right\":[{\"id\":\"dx\",\"label\":\"\",\"type\":\"foundation.electrical.electrical\"},{\"id\":\"bx\",\"label\":\"\",\"type\":\"foundation.electrical.electrical\"},{\"id\":\"sx\",\"label\":\"\",\"type\":\"foundation.electrical.electrical\"}],\"Top\":[]}"
  SPICE PMOS3 : ee_lib/Additional Components/SPICE Semiconductors/SPICE PMOS  LEVEL=3  AREA=1  SCALE=1  LENGTH=4 um  WIDTH=7 um  AD=0 m^2  AS=0 m^2  PD=0 m  PS=0 m  NRD=1  NRS=1  RD=0.01 Ohm  RS=1e-4 Ohm  RSH=NaN Ohm  VTO=0 V  KP=2e-5 A/V^2  GAMMA=0 V^0.50000  PHI=0.6 V  LAMBDA=0 1/V  IS=1e-14 A  N=1  JS=0 A/m^2  DELTA=0  VMAX=0 m/s  NFS=0 1/cm^2  ETA=0  THETA=0 1/V  KAPPA=0.2  Ci_param=ee.enum.intrinsicCapacitance.none  Cov_param=1  CGSO=0 F/m  CGDO=0 F/m  CGBO=0 F/m  C_param=1  CBD=0 F  CBS=0 F  PB=0.8 V  CJ=0 F/m^2  MJ=0.5  CJSW=0 F/m  MJSW=0.5  FC=0.5  IC_given=1  ICVDS=0 V  ICVGS=0 V  ICVBS=0 V  TOX=1e-7 m  LD=0 m  U0=600 cm^2/s/V  NSUB=NaN 1/cm^3  TPG=1  NSS=0 1/cm^2  XJ=0 m  T_param=1  TFIXED=300.15 K  TMEAS=300.15 K  TOFFSET=0 K  UEXP=0  UCRIT=1e+4 V/cm  NEFF=1  MTYPE=-1
      settings: InternalSimscapePortConfiguration="{\"Bottom\":[],\"Left\":[{\"id\":\"gx\",\"label\":\"\",\"type\":\"foundation.electrical.electrical\"}],\"Right\":[{\"id\":\"dx\",\"label\":\"\",\"type\":\"foundation.electrical.electrical\"},{\"id\":\"bx\",\"label\":\"\",\"type\":\"foundation.electrical.electrical\"},{\"id\":\"sx\",\"label\":\"\",\"type\":\"foundation.electrical.electrical\"}],\"Top\":[]}"
  SPICE PMOS4 : ee_lib/Additional Components/SPICE Semiconductors/SPICE PMOS  LEVEL=3  AREA=1  SCALE=1  LENGTH=5 um  WIDTH=4 um  AD=0 m^2  AS=0 m^2  PD=0 m  PS=0 m  NRD=1  NRS=1  RD=0.01 Ohm  RS=1e-4 Ohm  RSH=NaN Ohm  VTO=0 V  KP=2e-5 A/V^2  GAMMA=0 V^0.50000  PHI=0.6 V  LAMBDA=0 1/V  IS=1e-14 A  N=1  JS=0 A/m^2  DELTA=0  VMAX=0 m/s  NFS=0 1/cm^2  ETA=0  THETA=0 1/V  KAPPA=0.2  Ci_param=ee.enum.intrinsicCapacitance.none  Cov_param=1  CGSO=0 F/m  CGDO=0 F/m  CGBO=0 F/m  C_param=1  CBD=0 F  CBS=0 F  PB=0.8 V  CJ=0 F/m^2  MJ=0.5  CJSW=0 F/m  MJSW=0.5  FC=0.5  IC_given=1  ICVDS=0 V  ICVGS=0 V  ICVBS=0 V  TOX=1e-7 m  LD=0 m  U0=600 cm^2/s/V  NSUB=NaN 1/cm^3  TPG=1  NSS=0 1/cm^2  XJ=0 m  T_param=1  TFIXED=300.15 K  TMEAS=300.15 K  TOFFSET=0 K  UEXP=0  UCRIT=1e+4 V/cm  NEFF=1  MTYPE=-1
      settings: InternalSimscapePortConfiguration="{\"Bottom\":[],\"Left\":[{\"id\":\"gx\",\"label\":\"\",\"type\":\"foundation.electrical.electrical\"}],\"Right\":[{\"id\":\"dx\",\"label\":\"\",\"type\":\"foundation.electrical.electrical\"},{\"id\":\"bx\",\"label\":\"\",\"type\":\"foundation.electrical.electrical\"},{\"id\":\"sx\",\"label\":\"\",\"type\":\"foundation.electrical.electrical\"}],\"Top\":[]}"
  SPICE PMOS5 : ee_lib/Additional Components/SPICE Semiconductors/SPICE PMOS  LEVEL=3  AREA=1  SCALE=1  LENGTH=4 um  WIDTH=21 um  AD=0 m^2  AS=0 m^2  PD=0 m  PS=0 m  NRD=1  NRS=1  RD=0.01 Ohm  RS=1e-4 Ohm  RSH=NaN Ohm  VTO=0 V  KP=2e-5 A/V^2  GAMMA=0 V^0.50000  PHI=0.6 V  LAMBDA=0 1/V  IS=1e-14 A  N=1  JS=0 A/m^2  DELTA=0  VMAX=0 m/s  NFS=0 1/cm^2  ETA=0  THETA=0 1/V  KAPPA=0.2  Ci_param=ee.enum.intrinsicCapacitance.none  Cov_param=1  CGSO=0 F/m  CGDO=0 F/m  CGBO=0 F/m  C_param=1  CBD=0 F  CBS=0 F  PB=0.8 V  CJ=0 F/m^2  MJ=0.5  CJSW=0 F/m  MJSW=0.5  FC=0.5  IC_given=1  ICVDS=0 V  ICVGS=0 V  ICVBS=0 V  TOX=1e-7 m  LD=0 m  U0=600 cm^2/s/V  NSUB=NaN 1/cm^3  TPG=1  NSS=0 1/cm^2  XJ=0 m  T_param=1  TFIXED=300.15 K  TMEAS=300.15 K  TOFFSET=0 K  UEXP=0  UCRIT=1e+4 V/cm  NEFF=1  MTYPE=-1
      settings: InternalSimscapePortConfiguration="{\"Bottom\":[],\"Left\":[{\"id\":\"gx\",\"label\":\"\",\"type\":\"foundation.electrical.electrical\"}],\"Right\":[{\"id\":\"dx\",\"label\":\"\",\"type\":\"foundation.electrical.electrical\"},{\"id\":\"bx\",\"label\":\"\",\"type\":\"foundation.electrical.electrical\"},{\"id\":\"sx\",\"label\":\"\",\"type\":\"foundation.electrical.electrical\"}],\"Top\":[]}"
  SPICE PMOS6 : ee_lib/Additional Components/SPICE Semiconductors/SPICE PMOS  LEVEL=3  AREA=1  SCALE=1  LENGTH=4 um  WIDTH=7 um  AD=0 m^2  AS=0 m^2  PD=0 m  PS=0 m  NRD=1  NRS=1  RD=0.01 Ohm  RS=1e-4 Ohm  RSH=NaN Ohm  VTO=0 V  KP=2e-5 A/V^2  GAMMA=0 V^0.50000  PHI=0.6 V  LAMBDA=0 1/V  IS=1e-14 A  N=1  JS=0 A/m^2  DELTA=0  VMAX=0 m/s  NFS=0 1/cm^2  ETA=0  THETA=0 1/V  KAPPA=0.2  Ci_param=ee.enum.intrinsicCapacitance.none  Cov_param=1  CGSO=0 F/m  CGDO=0 F/m  CGBO=0 F/m  C_param=1  CBD=0 F  CBS=0 F  PB=0.8 V  CJ=0 F/m^2  MJ=0.5  CJSW=0 F/m  MJSW=0.5  FC=0.5  IC_given=1  ICVDS=0 V  ICVGS=0 V  ICVBS=0 V  TOX=1e-7 m  LD=0 m  U0=600 cm^2/s/V  NSUB=NaN 1/cm^3  TPG=1  NSS=0 1/cm^2  XJ=0 m  T_param=1  TFIXED=300.15 K  TMEAS=300.15 K  TOFFSET=0 K  UEXP=0  UCRIT=1e+4 V/cm  NEFF=1  MTYPE=-1
      settings: InternalSimscapePortConfiguration="{\"Bottom\":[],\"Left\":[{\"id\":\"gx\",\"label\":\"\",\"type\":\"foundation.electrical.electrical\"}],\"Right\":[{\"id\":\"dx\",\"label\":\"\",\"type\":\"foundation.electrical.electrical\"},{\"id\":\"bx\",\"label\":\"\",\"type\":\"foundation.electrical.electrical\"},{\"id\":\"sx\",\"label\":\"\",\"type\":\"foundation.electrical.electrical\"}],\"Top\":[]}"
  SPICE PMOS7 : ee_lib/Additional Components/SPICE Semiconductors/SPICE PMOS  LEVEL=3  AREA=1  SCALE=1  LENGTH=4 um  WIDTH=17 um  AD=0 m^2  AS=0 m^2  PD=0 m  PS=0 m  NRD=1  NRS=1  RD=0.01 Ohm  RS=1e-4 Ohm  RSH=NaN Ohm  VTO=0 V  KP=2e-5 A/V^2  GAMMA=0 V^0.50000  PHI=0.6 V  LAMBDA=0 1/V  IS=1e-14 A  N=1  JS=0 A/m^2  DELTA=0  VMAX=0 m/s  NFS=0 1/cm^2  ETA=0  THETA=0 1/V  KAPPA=0.2  Ci_param=ee.enum.intrinsicCapacitance.none  Cov_param=1  CGSO=0 F/m  CGDO=0 F/m  CGBO=0 F/m  C_param=1  CBD=0 F  CBS=0 F  PB=0.8 V  CJ=0 F/m^2  MJ=0.5  CJSW=0 F/m  MJSW=0.5  FC=0.5  IC_given=1  ICVDS=0 V  ICVGS=0 V  ICVBS=0 V  TOX=1e-7 m  LD=0 m  U0=600 cm^2/s/V  NSUB=NaN 1/cm^3  TPG=1  NSS=0 1/cm^2  XJ=0 m  T_param=1  TFIXED=300.15 K  TMEAS=300.15 K  TOFFSET=0 K  UEXP=0  UCRIT=1e+4 V/cm  NEFF=1  MTYPE=-1
      settings: InternalSimscapePortConfiguration="{\"Bottom\":[],\"Left\":[{\"id\":\"gx\",\"label\":\"\",\"type\":\"foundation.electrical.electrical\"}],\"Right\":[{\"id\":\"dx\",\"label\":\"\",\"type\":\"foundation.electrical.electrical\"},{\"id\":\"bx\",\"label\":\"\",\"type\":\"foundation.electrical.electrical\"},{\"id\":\"sx\",\"label\":\"\",\"type\":\"foundation.electrical.electrical\"}],\"Top\":[]}"
  Subsystem2 : Subsystem
  Subsystem3 : Subsystem
  V1 : PMIOPort  Side=Left
  In : PMIOPort  Port=2  Side=Left
  M16 : PMIOPort  Port=3  Side=Right
  V1_ : PMIOPort  Port=4  Side=Left
  out : PMIOPort  Port=5  Side=Left
  V3 : PMIOPort  Port=6  Side=Left
  Itail : PMIOPort  Port=7  Side=Right
  "node " : PMIOPort  Port=8  Side=Left
  connections:
  Electrical Reference12/LConn1 -- DC Voltage Source5/RConn1
  Electrical Reference13/LConn1 -- DC Voltage Source7/RConn1
  SPICE NMOS4/LConn1 -- V1_/RConn1
  Subsystem2/RConn1 -- Subsystem3/LConn1
  SPICE NMOS10/RConn1 -- SPICE NMOS8/RConn3 -- SPICE NMOS9/RConn3
  DC Voltage Source7/LConn1 -- SPICE NMOS6/RConn2 -- SPICE NMOS7/RConn2
  SPICE NMOS9/RConn1 -- SPICE NMOS8/RConn1 -- SPICE NMOS6/LConn1 -- SPICE PMOS6/RConn3 -- Subsystem3/RConn1 -- "node "/RConn1 -- SPICE NMOS4/RConn3 -- SPICE PMOS4/RConn1
  SPICE NMOS7/LConn1 -- SPICE NMOS7/RConn1 -- SPICE PMOS7/RConn3 -- SPICE NMOS10/LConn1
  SPICE PMOS3/RConn3 -- SPICE PMOS6/RConn1
  DC Voltage Source8/LConn1 -- SPICE PMOS5/RConn2 -- SPICE PMOS6/RConn2 -- SPICE PMOS3/RConn2 -- SPICE PMOS7/RConn2
  Electrical Reference14/LConn1 -- DC Voltage Source8/RConn1
  Electrical Reference9/LConn1 -- DC Voltage Source4/RConn1
  SPICE PMOS4/LConn1 -- V1/RConn1
  SPICE PMOS3/LConn1 -- M16/RConn1 -- SPICE PMOS5/LConn1
  In/RConn1 -- SPICE PMOS4/RConn3 -- SPICE NMOS4/RConn1
  Electrical Reference17/LConn1 -- DC Voltage Source6/RConn1 -- DC Voltage Source12/RConn1
  SPICE NMOS8/RConn2 -- SPICE NMOS9/RConn2 -- SPICE NMOS10/RConn2 -- DC Voltage Source5/LConn1
  DC Voltage Source12/LConn1 -- SPICE PMOS4/RConn2
  V3/RConn1 -- SPICE NMOS8/LConn1
  DC Voltage Source6/LConn1 -- SPICE NMOS4/RConn2
  SPICE PMOS5/RConn1 -- SPICE PMOS3/RConn1 -- DC Voltage Source4/LConn1
  Subsystem2/LConn1 -- out/RConn1
  SPICE NMOS7/RConn3 -- SPICE NMOS10/RConn3 -- Electrical Reference10/LConn1
  SPICE NMOS6/RConn1 -- SPICE PMOS7/RConn1 -- SPICE PMOS6/LConn1 -- SPICE PMOS5/RConn3
  SPICE PMOS7/LConn1 -- SPICE NMOS9/LConn1 -- Itail/RConn1 -- SPICE NMOS6/RConn3
